simulink model "dc_p_control"  (R2024b)
settings: Solver=VariableStepAuto  StartTime=0.0  StopTime=10.0  RelTol=1e-3
undefined symbols (not defined in the file): K
libraries: cstblocks x1
settings Model: Creator=martinhaugen  LastModifiedBy=martinhaugen

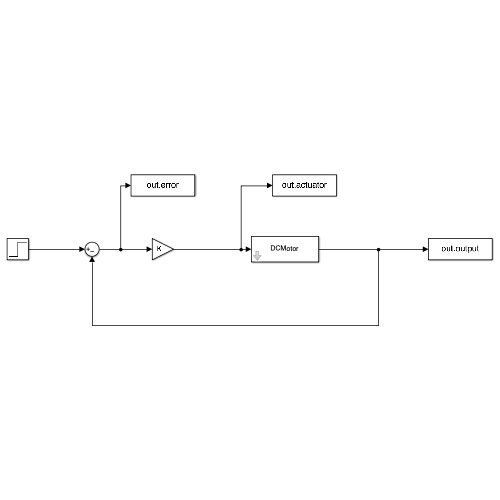
[thumbnail: Simulink's stored preview of the top-level diagram]
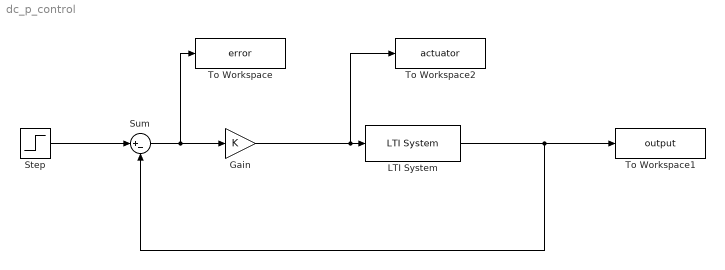
== system dc_p_control ==
  Gain : Gain  Gain=K
  LTI System : cstblocks/LTI System  sys=DCMotor  IC=[]  PadeOrder=0
  Step : Step  Time=0  SampleTime=0
  Sum : Sum  Inputs=|+-
  To Workspace : ToWorkspace  VariableName=error  SampleTime=-1
  To Workspace1 : ToWorkspace  VariableName=output  SampleTime=-1
  To Workspace2 : ToWorkspace  VariableName=actuator  SampleTime=-1
  wires:
  Gain/1 -> To Workspace2/1, LTI System/1
  Step/1 -> Sum/1
  Sum/1 -> To Workspace/1, Gain/1
  LTI System/1 -> To Workspace1/1, Sum/2
